simulink model "bpsk_pulse_generator"  (R2018a)
settings: Solver=VariableStepAuto  StartTime=0.0  StopTime=4  RelTol=1e-3
libraries: dsparch4 x1
settings Model: Creator=hp  LastModifiedBy=hp

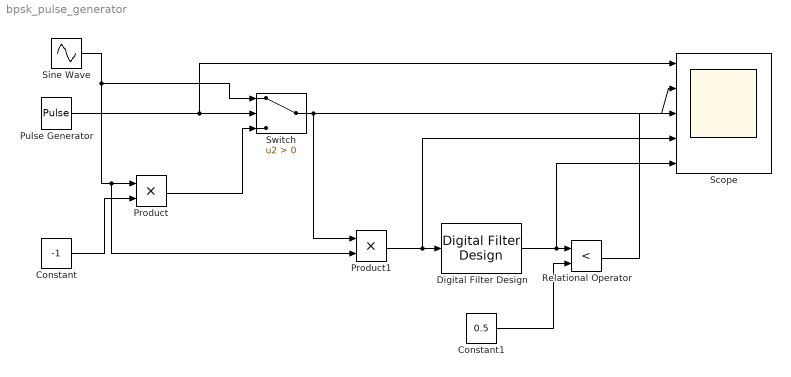
== system bpsk_pulse_generator ==
  Constant : Constant  Value=-1
  Constant1 : Constant  Value=0.5
  Digital Filter Design : dsparch4/Digital Filter Design  mwdsp_browser_bugfix_var=off
  Product : Product
  Product1 : Product
  Pulse Generator : DiscretePulseGenerator  PulseType=Time based  PulseWidth=50
  Relational Operator : RelationalOperator  Operator=<  OutDataTypeStr=boolean  RndMeth=Simplest
  Scope : Scope  NumInputPorts=5
  Sine Wave : Sin  Amplitude=2  Frequency=2*pi*4  SampleTime=0.01
  Switch : Switch  Criteria=u2 > Threshold
  wires:
  Sine Wave/1 -> Product1/2, Product/1, Switch/1
  Pulse Generator/1 -> Scope/1, Switch/2
  Product/1 -> Switch/3
  Constant/1 -> Product/2
  Switch/1 -> Product1/1, Scope/2
  Product1/1 -> Scope/4, Digital Filter Design/1
  Digital Filter Design/1 -> Scope/5, Relational Operator/1
  Constant1/1 -> Relational Operator/2
  Relational Operator/1 -> Scope/3
